simulink model "dc"  (R2022a)
settings: Solver=VariableStepAuto  StartTime=0.0  StopTime=12  RelTol=1e-3
libraries: spsDCVoltageSourceLib x2, spsDCMachineLib x1, spspowerguiLib x1
settings Model: SnapshotInterval=5  Creator=nivyachoudhary  LastModifiedBy=nivyachoudhary

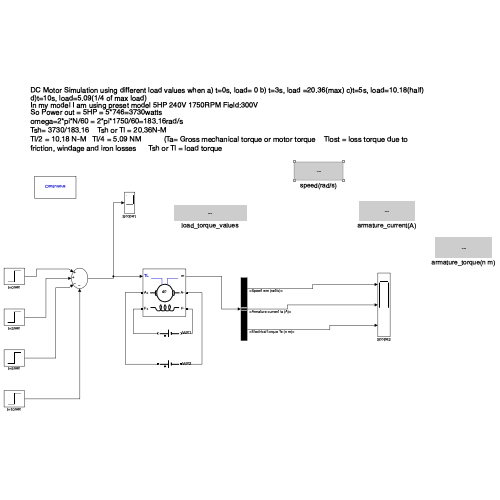
[thumbnail: Simulink's stored preview of the top-level diagram]
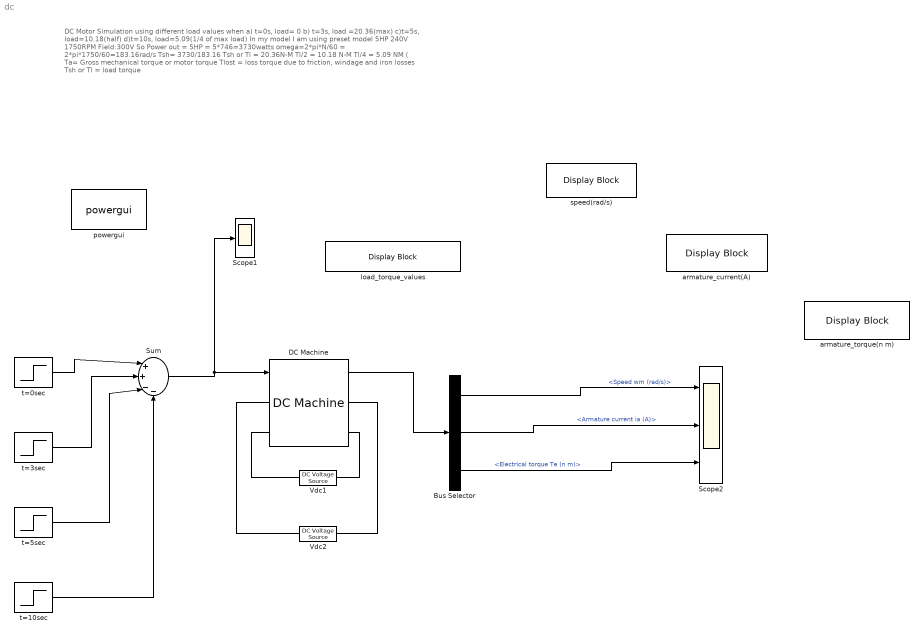
== system dc ==
  note: DC Motor Simulation using different load values when a) t=0s, load= 0 b) t=3s, load =20.36(max) c)t=5s, load=10.18(half) d)t=10s, load=5.09(1/4 of max load)
      | In my model I am using preset model 5HP 240V 1750RPM Field:300V
      | So Power out = 5HP = 5*746=3730watts
      | omega=2*pi*N/60 = 2*pi*1750/60=183.16rad/s
      | Tsh= 3730/183.16 Tsh or Tl = 20.36N-M
      | Tl/2 = 10.18 N-M Tl/4 = 5.09 NM ( Ta= Gross mechanical torque or motor torque Tlost = loss torque due to friction, windage and iron losses Tsh or Tl = load torque
  Bus Selector : BusSelector  OutputSignals=Speed wm (rad/s),Armature current ia (A),Electrical torque Te (n m)
  DC Machine : spsDCMachineLib/DC Machine  PresetModel=01: 5HP 240V 1750RPM Field:300V  MechanicalLoad=Torque TL  FieldType=Wound  ShowDetailedParameters=on  MeasurementBus=off  RLa=[2.581 0.028]  RLf=[281.2 156]  Laf=0.9483  MachineConstant=Torque constant (N.m/A)  Ke=1.8  Kt=1.8  J=0.02215  Bm=0.002953  Tf=0.5161  w0=1  Ifinit=1.06685633001422  TsPowergui=0  TsBlock=-1
  Scope1 : Scope
  Scope2 : Scope  NumInputPorts=3
  Sum : Sum  Inputs=|++--
  Vdc1 : spsDCVoltageSourceLib/DC Voltage Source  Amplitude=300  Measurements=None
  Vdc2 : spsDCVoltageSourceLib/DC Voltage Source  Amplitude=240  Measurements=None
  armature_current(A) : DisplayBlock  LabelPosition=Hide  Transparency=1
  armature_torque(n m) : DisplayBlock  LabelPosition=Hide  Transparency=1
  load_torque_values : DisplayBlock  LabelPosition=Hide  Transparency=1
  powergui : spspowerguiLib/powergui  Priority=1  SimulationMode=Continuous  SampleTime=50e-6  frequency=60  Iterations=50  frequencyindice=0  Pbase=100e6  ErrMax=1e-4  UnitsV=kV  UnitsW=MW  buscounter=0  FunctionMessages=off  echomessages=off  EnableUseOfTLC=off  CurrentSourceSwitches=off  DisableSnubberDevices=off  DisableRonSwitches=off  DisableVfSwitches=off  DisplayEquations=off  AutomaticDiscreteSolvers=off  SolverType=Tustin/Backward Euler (TBE)  Interpol=off  ExternalGateDelay=off  methode=off  Ts=100  x0status=blocks  SPID=on  SwTol=0  HookPort=off  NonlinearTolerance=1e-4  nMaxIteration=100  ContinueOnMaxIteration=off  RestoreLinks=warning  ResistiveCurrentMeasurement=off  Frange=[0:2:500]  Ylog=off  Xlog=on  ShowGrid=off  save=off  variable=ZData  structure=0  ZoomFFT=off  StartTime=0.0  cycles=1  DisplayStyle=1  fundamental=60  FreqAxis=off  MaxFrequency=1000  frequencyindicesteady=1  RmsSteady=1  display=off
  speed(rad/s) : DisplayBlock  LabelPosition=Hide  Transparency=1
  t=0sec : Step  Time=0  After=0  SampleTime=0
  t=10sec : Step  Time=10  After=5.09  SampleTime=0
  t=3sec : Step  Time=3  After=20.36  SampleTime=0
  t=5sec : Step  Time=5  After=10.18  SampleTime=0
  wires:
  DC Machine/1 -> Bus Selector/1
  Bus Selector/2 -> Scope2/2  "<Armature current ia (A)>"
  Bus Selector/3 -> Scope2/3  "<Electrical torque Te (n m)>"
  Sum/1 -> Scope1/1, DC Machine/1
  t=0sec/1 -> Sum/1
  t=3sec/1 -> Sum/2
  t=5sec/1 -> Sum/3
  t=10sec/1 -> Sum/4
  Bus Selector/1 -> Scope2/1  "<Speed wm (rad/s)>"
  connections:
  Vdc1/RConn1 -- DC Machine/LConn2
  Vdc1/LConn1 -- DC Machine/RConn2
  DC Machine/RConn1 -- Vdc2/LConn1
  Vdc2/RConn1 -- DC Machine/LConn1
